simulink model "lab1b"  (R2023a)
settings: Solver=VariableStepAuto  StartTime=0.0  StopTime=10.0  RelTol=1e-3
settings Model: Creator=CSE-LAB2-64  LastModifiedBy=CSE-LAB2-64

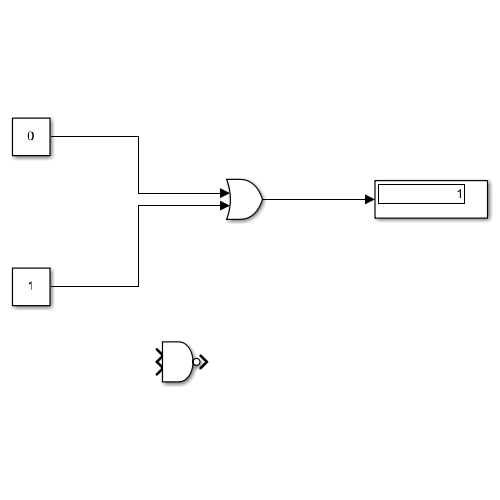
[thumbnail: Simulink's stored preview of the top-level diagram]
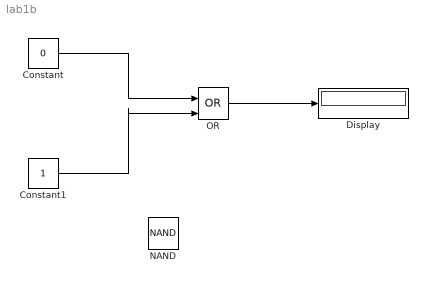
== system lab1b ==
  Constant : Constant  Value=0
  Constant1 : Constant
  Display : Display
  NAND : Logic  Operator=NAND  IconShape=distinctive  AllPortsSameDT=off  OutDataTypeStr=boolean
  OR : Logic  Operator=OR  IconShape=distinctive  AllPortsSameDT=off  OutDataTypeStr=boolean
  wires:
  Constant/1 -> OR/1
  Constant1/1 -> OR/2
  OR/1 -> Display/1
